simulink model "Tarea1"  (R2022a)
settings: Solver=VariableStepAuto  StartTime=0.0  StopTime=250  RelTol=1e-3
settings Model: Creator=bluep  LastModifiedBy=bluep

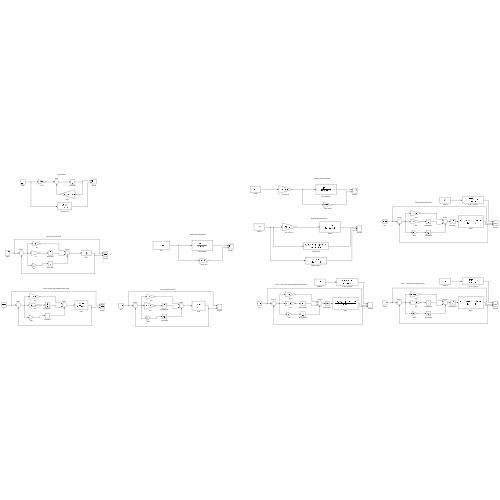
[thumbnail: Simulink's stored preview of the top-level diagram]
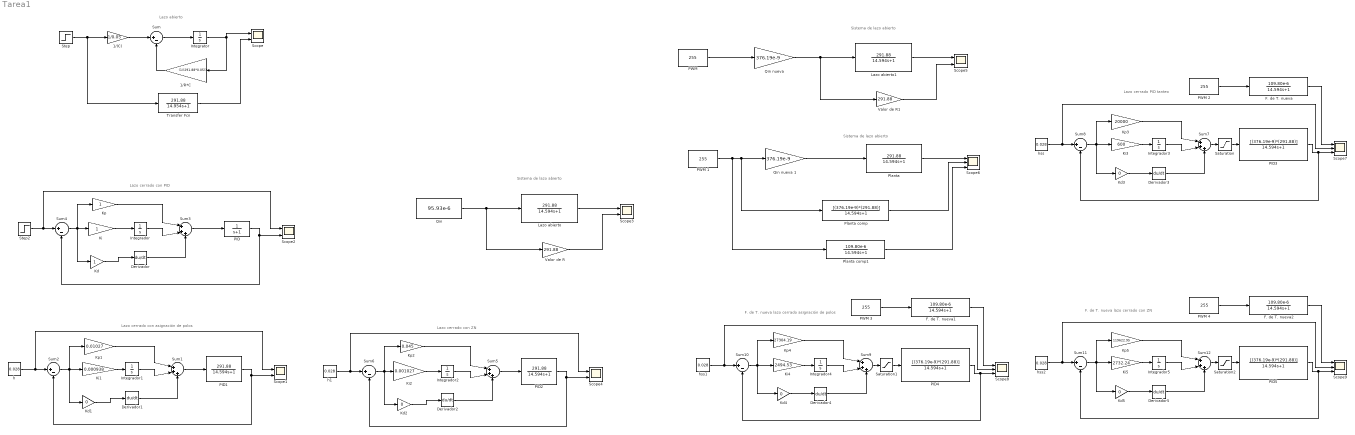
== system Tarea1 ==
  note: Sistema de lazo abierto
  note: Lazo cerrado con PID
  note: Lazo abierto
  note: Lazo cerrado con asignación de polos
  note: Lazo cerrado con ZN
  note: Sistema de lazo abierto
  note: Sistema de lazo abierto
  note: Lazo cerrado PID tanteo
  note: F. de T. nueva lazo cerrado asignación de polos
  note: F. de T. nueva lazo cerrado con ZN
  1/(C) : Gain  Gain=1/0.05
  1/R*C : Gain  Gain=(1/(291.88*0.05))
  Derivador{,1..5} (6 alike) : Derivative
  F. de T. nueva : TransferFcn  Numerator=[109.80e-6]  Denominator=[14.594 1]
  F. de T. nueva1 : TransferFcn  Numerator=[109.80e-6]  Denominator=[14.594 1]
  F. de T. nueva2 : TransferFcn  Numerator=[109.80e-6]  Denominator=[14.594 1]
  Integrador{,1..5} (6 alike) : Integrator
  Integrator : Integrator
  Kd : Gain
  Kd{1..5} (5 alike) : Gain  Gain=0
  Ki : Gain
  Ki1 : Gain  Gain=0.000938
  Ki2 : Gain  Gain=0.001027
  Ki3 : Gain  Gain=600
  Ki4 : Gain  Gain=2494.53
  Ki5 : Gain  Gain=2732.24
  Kp : Gain
  Kp1 : Gain  Gain=0.01027
  Kp2 : Gain  Gain=0.045
  Kp3 : Gain  Gain=20000
  Kp4 : Gain  Gain=27304.19
  Kp5 : Gain  Gain=119622.95
  Lazo abierto : TransferFcn  Numerator=[291.88]  Denominator=[14.594 1]
  Lazo abierto1 : TransferFcn  Numerator=[291.88]  Denominator=[14.594 1]
  PID : TransferFcn  Denominator=[1 1]
  PID1 : TransferFcn  Numerator=291.88  Denominator=[14.594 1]
  PID2 : TransferFcn  Numerator=[291.88]  Denominator=[14.594 1]
  PID3 : TransferFcn  Numerator=[(376.19e-9)*(291.88)]  Denominator=[14.594 1]
  PID4 : TransferFcn  Numerator=[(376.19e-9)*(291.88)]  Denominator=[14.594 1]
  PID5 : TransferFcn  Numerator=[(376.19e-9)*(291.88)]  Denominator=[14.594 1]
  PWM : Constant  Value=255
  PWM {1..4} (4 alike) : Constant  Value=255
  Planta : TransferFcn  Numerator=[291.88]  Denominator=[14.594 1]
  Planta comp : TransferFcn  Numerator=[(376.19e-9)*(291.88)]  Denominator=[14.594 1]
  Planta comp1 : TransferFcn  Numerator=[109.80e-6]  Denominator=[14.594 1]
  Qin : Constant  Value=95.93e-6
  Qin nueva : Gain  Gain=376.19e-9
  Qin nueva 1 : Gain  Gain=376.19e-9
  Saturation : Saturate  UpperLimit=255  LowerLimit=0
  Saturation1 : Saturate  UpperLimit=255  LowerLimit=0
  Saturation2 : Saturate  UpperLimit=255  LowerLimit=0
  Scope{,1..5} (6 alike) : Scope  NumInputPorts=2
  Scope{6..9} (4 alike) : Scope  NumInputPorts=3
  Step : Step  Time=0  SampleTime=0
  Step2 : Step  Time=0  SampleTime=0
  Sum{,2,4,6,8,10..11} (7 alike) : Sum  Inputs=|+-
  Sum{1,3,5,7,9,12} (6 alike) : Sum  Inputs=|+++
  Transfer Fcn : TransferFcn  Numerator=[291.88]  Denominator=[14.954 1]
  Valor de R : Gain  Gain=291.88
  Valor de R1 : Gain  Gain=291.88
  h : Constant  Value=0.028
  h1 : Constant  Value=0.028
  hss : Constant  Value=0.028
  hss1 : Constant  Value=0.028
  hss2 : Constant  Value=0.028
  wires:
  Step/1 -> Transfer Fcn/1, 1/(C)/1
  1/(C)/1 -> Sum/1
  Sum/1 -> Integrator/1
  Integrator/1 -> 1/R*C/1, Scope/1
  1/R*C/1 -> Sum/2
  Transfer Fcn/1 -> Scope/2
  Ki/1 -> Integrador/1
  Kp/1 -> Sum3/1
  Integrador/1 -> Sum3/2
  Derivador/1 -> Sum3/3
  Kd/1 -> Derivador/1
  Sum4/1 -> Kd/1, Kp/1, Ki/1
  Sum3/1 -> PID/1
  PID/1 -> Scope2/2, Sum4/2
  Step2/1 -> Scope2/1, Sum4/1
  Qin/1 -> Valor de R/1, Lazo abierto/1
  Valor de R/1 -> Scope3/2
  Lazo abierto/1 -> Scope3/1
  Sum1/1 -> PID1/1
  h/1 -> Scope1/1, Sum2/1
  Derivador1/1 -> Sum1/3
  Ki1/1 -> Integrador1/1
  Kp1/1 -> Sum1/1
  PID1/1 -> Scope1/2, Sum2/2
  Sum2/1 -> Kd1/1, Kp1/1, Ki1/1
  Kd1/1 -> Derivador1/1
  Integrador1/1 -> Sum1/2
  PID2/1 -> Scope4/2, Sum6/2
  Kp2/1 -> Sum5/1
  Ki2/1 -> Integrador2/1
  Sum6/1 -> Kp2/1, Ki2/1, Kd2/1
  Integrador2/1 -> Sum5/2
  h1/1 -> Scope4/1, Sum6/1
  Kd2/1 -> Derivador2/1
  Sum5/1 -> PID2/1
  Derivador2/1 -> Sum5/3
  Valor de R1/1 -> Scope5/2
  Lazo abierto1/1 -> Scope5/1
  PWM/1 -> Qin nueva/1
  Qin nueva/1 -> Valor de R1/1, Lazo abierto1/1
  Qin nueva 1/1 -> Planta/1
  Planta/1 -> Scope6/1
  PWM 1/1 -> Planta comp1/1, Planta comp/1, Qin nueva 1/1
  Planta comp/1 -> Scope6/2
  Planta comp1/1 -> Scope6/3
  Kd3/1 -> Derivador3/1
  Sum8/1 -> Kd3/1, Kp3/1, Ki3/1
  Integrador3/1 -> Sum7/2
  Ki3/1 -> Integrador3/1
  Kp3/1 -> Sum7/1
  Derivador3/1 -> Sum7/3
  PID3/1 -> Scope7/3, Sum8/2
  hss/1 -> Scope7/2, Sum8/1
  Sum7/1 -> Saturation/1
  Saturation/1 -> PID3/1
  PWM 2/1 -> F. de T. nueva/1
  F. de T. nueva/1 -> Scope7/1
  PWM 3/1 -> F. de T. nueva1/1
  hss1/1 -> Scope8/2, Sum10/1
  Saturation1/1 -> PID4/1
  F. de T. nueva1/1 -> Scope8/1
  Sum9/1 -> Saturation1/1
  Sum10/1 -> Kd4/1, Kp4/1, Ki4/1
  Integrador4/1 -> Sum9/2
  Ki4/1 -> Integrador4/1
  PID4/1 -> Scope8/3, Sum10/2
  Derivador4/1 -> Sum9/3
  Kp4/1 -> Sum9/1
  Kd4/1 -> Derivador4/1
  Kd5/1 -> Derivador5/1
  PID5/1 -> Scope9/3, Sum11/2
  Derivador5/1 -> Sum12/3
  Integrador5/1 -> Sum12/2
  Ki5/1 -> Integrador5/1
  Sum11/1 -> Kd5/1, Kp5/1, Ki5/1
  Sum12/1 -> Saturation2/1
  Saturation2/1 -> PID5/1
  F. de T. nueva2/1 -> Scope9/1
  hss2/1 -> Scope9/2, Sum11/1
  Kp5/1 -> Sum12/1
  PWM 4/1 -> F. de T. nueva2/1
